simulink model "ES249A_MotAgCorrln"  (R2013b)
settings: Solver=FixedStepDiscrete  SolverMode=SingleTasking  StartTime=0.0  StopTime=1  FixedStep=0.002  RelTol=1e-3
undefined symbols (not defined in the file): FLTINJ_MOTAGCORRLN_MOTAGIDPTSIG, HALFREV_MOTREV_U0P16, MOTAGACORRLNST_CNT_U08, MotAgAMotAgBCorrln, MotAgAMotAgCCorrln, MOTAGBCORRLNST_CNT_U08, MotAgBMotAgCCorrln, MOTAGCCORRLNST_CNT_U08, MOTAGCORRLNERRTHD_MOTREVELEC_U0P16, MOTAGCORRLNNTCFAILSTEP_CNT_U16, MOTAGCORRLNNTCPASSSTEP_CNT_U16, MOTAGMAXSTALLCNTR_CNT_U08, MotAgMeclCorrlnSt, MotAgMeclIdptSig, NtcSts1, sigbuilder_block, SysGlbPrmMotPoleCnt
libraries: simulink x5
(part 4 of 4)

== stateflow chart ES249A_MotAgCorrln/MotAgCorrln/MotAgCorrlnPer1/MotAgA vs MotAgB/SetNtcSts/ISO Fault Debounce Design NOT TO BE IMPLEMENTED IN THIS FDD USED ONLY FOR SIMULATION PURPOSES ==
  note: NTCSTS_PASSD           (0)
      | NTCSTS_FAILD             (1)
      | NTCSTS_PREPASSD   (2)
      | NTCSTS_PREFAILD     (3)
      |
      | SIGQLFR_NORES        (0)
      | SIGQLFR_PASSD         (1)
      | SIGQLFR_FAILD           (2)
  note: Nstep Loop
  note: Pstep Loop
  note: 
  (default) -> (junction 89)
  (junction 89) -> (junction 95) [order 1] : [NtcSts == 3]
  (junction 89) -> (junction 93) [order 2] : [ NtcSts == 2]
  (junction 93) -> (junction 230) [order 2] : {
      | ErrAcc = ErrAcc - DebStep;
      | }
  (junction 95) -> (junction 213) [order 1] : [ErrAcc <=0]
      | {
      | ErrAcc = DebStep;
      | }
  (junction 95) -> (junction 103) [order 2]
  (junction 89) -> (junction 221) [order 3] : [(NtcSts == 0) | ...
      | (NtcSts == 1)]
  (junction 93) -> (junction 123) [order 1] : [(ErrAcc - DebStep) <= -32768]
      | {
      | ErrAcc = -32768;
      | Qualifier = 1;
      | }
  (junction 230) -> (junction 231)
  (junction 213) -> (junction 216)
  (junction 103) -> (junction 216) [order 2] : {
      | ErrAcc = ErrAcc + DebStep;
      | }
  (junction 221) -> (junction 222) [order 2] : [NtcSts == 0]
      | {
      | ErrAcc = -32768;
      | Qualifier=1;
      | }
  (junction 216) -> (junction 214)
  (junction 103) -> (junction 220) [order 1] : [(ErrAcc + DebStep) >=32767]
      | {
      | ErrAcc = 32767;
      | Qualifier =2;
      | }
  (junction 221) -> (junction 212) [order 1] : [NtcSts == 1]
      | {
      | ErrAcc = 32767;
      | Qualifier =2;
      |  }
  (junction 222) -> (junction 225)
  (junction 225) -> (junction 212)
  (junction 212) -> (junction 141)
  (junction 214) -> (junction 220)
  (junction 220) -> (junction 141)
  (junction 123) -> (junction 141)
  (junction 231) -> (junction 123)
  (junction 141) -> (junction 159)
  (junction 159) -> (junction 235) [order 2]
  (junction 235) -> (junction 236)
  (junction 159) -> (junction 234) [order 1] : [SvcClr ==1]
      | {
      | ErrAcc = 0;
      | Qualifier =0;
      | }
  (junction 236) -> (junction 234)
  data: NtcSts input uint8; Qualifier output uint8; DebStep input uint16; ErrAcc output int16; SvcClr input

== matlab function ES249A_MotAgCorrln/MotAgCorrln/MotAgCorrlnPer1/TestOk ==
  data: MotAgAvsMotAgB input boolean; MotAgAOk output boolean; MotAgAvsMotAgC input boolean; MotAgBvsMotAgC input boolean; MotAgBOk output boolean; MotAgCOk output boolean
function [MotAgAOk, MotAgBOk, MotAgCOk] = fcn(MotAgAvsMotAgB, MotAgAvsMotAgC, MotAgBvsMotAgC)

aVarTruthTableCondition_1 = false;
aVarTruthTableCondition_2 = false;
aVarTruthTableCondition_3 = false;


% MotAgAvsMotAgB TestOk

aVarTruthTableCondition_1 = logical(MotAgAvsMotAgB == 1);

% MotAgAvsMotAgC TestOk

aVarTruthTableCondition_2 = logical(MotAgAvsMotAgC == 1);

% MotAgBvsMotAgC TestOk

aVarTruthTableCondition_3 = logical(MotAgBvsMotAgC == 1);

if (aVarTruthTableCondition_1 && aVarTruthTableCondition_2 && aVarTruthTableCondition_3)
    aFcnTruthTableAction_1();
elseif (aVarTruthTableCondition_1 && aVarTruthTableCondition_2 && ~aVarTruthTableCondition_3)
    aFcnTruthTableAction_1();
elseif (aVarTruthTableCondition_1 && ~aVarTruthTableCondition_2 && aVarTruthTableCondition_3)
    aFcnTruthTableAction_1();
elseif (aVarTruthTableCondition_1 && ~aVarTruthTableCondition_2 && ~aVarTruthTableCondition_3)
    aFcnTruthTableAction_2();
elseif (~aVarTruthTableCondition_1 && aVarTruthTableCondition_2 && aVarTruthTableCondition_3)
    aFcnTruthTableAction_1();
elseif (~aVarTruthTableCondition_1 && aVarTruthTableCondition_2 && ~aVarTruthTableCondition_3)
    aFcnTruthTableAction_3();
elseif (~aVarTruthTableCondition_1 && ~aVarTruthTableCondition_2 && aVarTruthTableCondition_3)
    aFcnTruthTableAction_4();
else % Default
    aFcnTruthTableAction_5();
end

function aFcnTruthTableAction_1()

% All good

MotAgAOk = true;
MotAgBOk = true;
MotAgCOk = true;

function aFcnTruthTableAction_2()

% 1 and 2 good

MotAgAOk = true;
MotAgBOk = true;
MotAgCOk = false;

function aFcnTruthTableAction_3()

% 1 and 3 good

MotAgAOk = true;
MotAgBOk = false;
MotAgCOk = true;

function aFcnTruthTableAction_4()

% 2 and 3 good

MotAgAOk = false;
MotAgBOk = true;
MotAgCOk = true;

function aFcnTruthTableAction_5()

% Default (none good)

MotAgAOk = false;
MotAgBOk = false;
MotAgCOk = false;

== stateflow chart ES249A_MotAgCorrln/MotAgCorrln/MotAgCorrlnPer1/MotAgA vs MotAgC/SetNtcSts/ISO Fault Debounce Design NOT TO BE IMPLEMENTED IN THIS FDD USED ONLY FOR SIMULATION PURPOSES ==
  note: NTCSTS_PASSD           (0)
      | NTCSTS_FAILD             (1)
      | NTCSTS_PREPASSD   (2)
      | NTCSTS_PREFAILD     (3)
      |
      | SIGQLFR_NORES        (0)
      | SIGQLFR_PASSD         (1)
      | SIGQLFR_FAILD           (2)
  note: Nstep Loop
  note: Pstep Loop
  note: 
  (default) -> (junction 89)
  (junction 89) -> (junction 95) [order 1] : [NtcSts == 3]
  (junction 89) -> (junction 93) [order 2] : [ NtcSts == 2]
  (junction 93) -> (junction 230) [order 2] : {
      | ErrAcc = ErrAcc - DebStep;
      | }
  (junction 95) -> (junction 213) [order 1] : [ErrAcc <=0]
      | {
      | ErrAcc = DebStep;
      | }
  (junction 95) -> (junction 103) [order 2]
  (junction 89) -> (junction 221) [order 3] : [(NtcSts == 0) | ...
      | (NtcSts == 1)]
  (junction 93) -> (junction 123) [order 1] : [(ErrAcc - DebStep) <= -32768]
      | {
      | ErrAcc = -32768;
      | Qualifier = 1;
      | }
  (junction 230) -> (junction 231)
  (junction 213) -> (junction 216)
  (junction 103) -> (junction 216) [order 2] : {
      | ErrAcc = ErrAcc + DebStep;
      | }
  (junction 221) -> (junction 222) [order 2] : [NtcSts == 0]
      | {
      | ErrAcc = -32768;
      | Qualifier=1;
      | }
  (junction 216) -> (junction 214)
  (junction 103) -> (junction 220) [order 1] : [(ErrAcc+DebStep) >=32767]
      | {
      | ErrAcc = 32767;
      | Qualifier =2;
      | }
  (junction 221) -> (junction 212) [order 1] : [NtcSts == 1]
      | {
      | ErrAcc = 32767;
      | Qualifier =2;
      |  }
  (junction 222) -> (junction 225)
  (junction 225) -> (junction 212)
  (junction 212) -> (junction 141)
  (junction 214) -> (junction 220)
  (junction 220) -> (junction 141)
  (junction 123) -> (junction 141)
  (junction 231) -> (junction 123)
  (junction 141) -> (junction 159)
  (junction 159) -> (junction 235) [order 2]
  (junction 235) -> (junction 236)
  (junction 159) -> (junction 234) [order 1] : [SvcClr ==1]
      | {
      | ErrAcc = 0;
      | Qualifier =0;
      | }
  (junction 236) -> (junction 234)
  data: NtcSts input uint8; Qualifier output uint8; DebStep input uint16; ErrAcc output int16; SvcClr input

== matlab function ES249A_MotAgCorrln/MotAgCorrln/MotAgCorrlnPer1/NotFailed ==
  data: MotAgAvsMotAgB input uint8; MotAgSigAvlA input boolean; MotAgANotFailed output boolean; MotAgAvsMotAgC input uint8; MotAgSigAvlB input boolean; MotAgBvsMotAgC input uint8; MotAgBNotFailed output boolean; MotAgCNotFailed output boolean; MotAgMeclIdptSig output uint8; MotAgSigAvlC input boolean
function [MotAgANotFailed, MotAgBNotFailed, MotAgCNotFailed, MotAgMeclIdptSig] = fcn(MotAgAvsMotAgB, MotAgSigAvlA, MotAgAvsMotAgC, MotAgSigAvlB, MotAgBvsMotAgC, MotAgSigAvlC)

aVarTruthTableCondition_1 = false;
aVarTruthTableCondition_2 = false;
aVarTruthTableCondition_3 = false;


% MotAgAvsMotAgB Not Failed

aVarTruthTableCondition_1 = logical(MotAgAvsMotAgB < 2);

% MotAgAvsMotAgC Not Failed

aVarTruthTableCondition_2 = logical(MotAgAvsMotAgC < 2);

% MotAgBvsMotAgC Not Failed

aVarTruthTableCondition_3 = logical(MotAgBvsMotAgC < 2);

if (aVarTruthTableCondition_1 && aVarTruthTableCondition_2 && aVarTruthTableCondition_3)
    aFcnTruthTableAction_1();
elseif (aVarTruthTableCondition_1 && aVarTruthTableCondition_2 && ~aVarTruthTableCondition_3)
    aFcnTruthTableAction_1();
elseif (aVarTruthTableCondition_1 && ~aVarTruthTableCondition_2 && aVarTruthTableCondition_3)
    aFcnTruthTableAction_1();
elseif (aVarTruthTableCondition_1 && ~aVarTruthTableCondition_2 && ~aVarTruthTableCondition_3)
    aFcnTruthTableAction_2();
elseif (~aVarTruthTableCondition_1 && aVarTruthTableCondition_2 && aVarTruthTableCondition_3)
    aFcnTruthTableAction_1();
elseif (~aVarTruthTableCondition_1 && aVarTruthTableCondition_2 && ~aVarTruthTableCondition_3)
    aFcnTruthTableAction_3();
elseif (~aVarTruthTableCondition_1 && ~aVarTruthTableCondition_2 && aVarTruthTableCondition_3)
    aFcnTruthTableAction_4();
else % Default
    aFcnTruthTableAction_5();
end

function aFcnTruthTableAction_1()

% All good

MotAgANotFailed = true;
MotAgBNotFailed = true;
MotAgCNotFailed = true;
MotAgMeclIdptSig=uint8(MotAgSigAvlA+MotAgSigAvlB+MotAgSigAvlC);

function aFcnTruthTableAction_2()

% 1 and 2 good

MotAgANotFailed = true;
MotAgBNotFailed = true;
MotAgCNotFailed = false;
MotAgMeclIdptSig = uint8(MotAgSigAvlA+MotAgSigAvlB);

function aFcnTruthTableAction_3()

% 1 and 3 good

MotAgANotFailed = true;
MotAgBNotFailed = false;
MotAgCNotFailed = true;
MotAgMeclIdptSig=uint8(MotAgSigAvlA+MotAgSigAvlC);

function aFcnTruthTableAction_4()

% 2 and 3 good

MotAgANotFailed = false;
MotAgBNotFailed = true;
MotAgCNotFailed = true;
MotAgMeclIdptSig=uint8(MotAgSigAvlB+MotAgSigAvlC);

function aFcnTruthTableAction_5()

% Default (none good)

MotAgANotFailed = false;
MotAgBNotFailed = false;
MotAgCNotFailed = false;
MotAgMeclIdptSig = uint8(0);

== stateflow chart ES249A_MotAgCorrln/MotAgCorrln/MotAgCorrlnPer1/MotAgB vs MotAgC/SetNtcSts/ISO Fault Debounce Design NOT TO BE IMPLEMENTED IN THIS FDD USED ONLY FOR SIMULATION PURPOSES ==
  note: NTCSTS_PASSD           (0)
      | NTCSTS_FAILD             (1)
      | NTCSTS_PREPASSD   (2)
      | NTCSTS_PREFAILD     (3)
      |
      | SIGQLFR_NORES        (0)
      | SIGQLFR_PASSD         (1)
      | SIGQLFR_FAILD           (2)
  note: Nstep Loop
  note: Pstep Loop
  note: 
  (default) -> (junction 89)
  (junction 89) -> (junction 95) [order 1] : [NtcSts == 3]
  (junction 89) -> (junction 93) [order 2] : [ NtcSts == 2]
  (junction 93) -> (junction 230) [order 2] : {
      | ErrAcc = ErrAcc - DebStep;
      | }
  (junction 95) -> (junction 213) [order 1] : [ErrAcc <=0]
      | {
      | ErrAcc = DebStep;
      | }
  (junction 95) -> (junction 103) [order 2]
  (junction 89) -> (junction 221) [order 3] : [(NtcSts == 0) | ...
      | (NtcSts == 1)]
  (junction 93) -> (junction 123) [order 1] : [(ErrAcc - DebStep) <= -32768]
      | {
      | ErrAcc = -32768;
      | Qualifier = 1;
      | }
  (junction 230) -> (junction 231)
  (junction 213) -> (junction 216)
  (junction 103) -> (junction 216) [order 2] : {
      | ErrAcc = ErrAcc + DebStep;
      | }
  (junction 221) -> (junction 222) [order 2] : [NtcSts == 0]
      | {
      | ErrAcc = -32768;
      | Qualifier=1;
      | }
  (junction 216) -> (junction 214)
  (junction 103) -> (junction 220) [order 1] : [(ErrAcc + DebStep) >=32767]
      | {
      | ErrAcc = 32767;
      | Qualifier =2;
      | }
  (junction 221) -> (junction 212) [order 1] : [NtcSts == 1]
      | {
      | ErrAcc = 32767;
      | Qualifier =2;
      |  }
  (junction 222) -> (junction 225)
  (junction 225) -> (junction 212)
  (junction 212) -> (junction 141)
  (junction 214) -> (junction 220)
  (junction 220) -> (junction 141)
  (junction 123) -> (junction 141)
  (junction 231) -> (junction 123)
  (junction 141) -> (junction 159)
  (junction 159) -> (junction 235) [order 2]
  (junction 235) -> (junction 236)
  (junction 159) -> (junction 234) [order 1] : [SvcClr ==1]
      | {
      | ErrAcc = 0;
      | Qualifier =0;
      | }
  (junction 236) -> (junction 234)
  data: NtcSts input uint8; Qualifier output uint8; DebStep input uint16; ErrAcc output int16; SvcClr input

== stateflow chart ES249A_MotAgCorrln/MotAgCorrln/MotAgCorrlnPer1/MtrAgC SigAvlCheck/CorrSigAvlChkRev1 ==
  note: SigAvl
      | False = 0
      | Pass = 1
  note: SigQlfr
      | 0 = No Result
      | 1 = Pass
      | 2 = Fail
  (default) -> (junction 2)
  (junction 2) -> (junction 4) [order 1] : [SigRollgCnt ==LstRollgCnt]
  (junction 4) -> (junction 7) [order 2] : {
      | StallCntOutp = LstStallCnt +1;
      | }
  (junction 2) -> (junction 3) [order 2]
  (junction 4) -> (junction 7) [order 1] : [LstStallCnt == 255]
      | {
      | StallCntOutp = 255;
      | }
  (junction 3) -> (junction 7) : {
      | StallCntOutp = 0;
      | }
  (junction 7) -> (junction 10)
  (junction 10) -> (junction 12) [order 1] : [StallCntOutp >=kMaxStallCnt]
  (junction 10) -> (junction 14) [order 2]
  (junction 12) -> (junction 17)
  (junction 14) -> (junction 17) [order 2]
  (junction 14) -> (junction 16) [order 1] : [SigQlfr<2]
  (junction 17) -> (junction 29) : {
      | SigAvl =0;
      | }
  (junction 16) -> (junction 29) : {
      | SigAvl = 1;
      | }
  data: SigRollgCnt input; SigQlfr input; kMaxStallCnt input; SigAvl output boolean; LstRollgCnt input uint8; LstStallCnt input uint8; StallCntOutp output uint8

== stateflow chart ES249A_MotAgCorrln/MotAgCorrln/MotAgCorrlnPer1/MtrAgB SigAvlCheck/CorrSigAvlChkRev1 ==
  note: SigAvl
      | False = 0
      | Pass = 1
  note: SigQlfr
      | 0 = No Result
      | 1 = Pass
      | 2 = Fail
  (default) -> (junction 2)
  (junction 2) -> (junction 4) [order 1] : [SigRollgCnt ==LstRollgCnt]
  (junction 4) -> (junction 7) [order 2] : {
      | StallCntOutp = LstStallCnt +1;
      | }
  (junction 2) -> (junction 3) [order 2]
  (junction 4) -> (junction 7) [order 1] : [LstStallCnt == 255]
      | {
      | StallCntOutp = 255;
      | }
  (junction 3) -> (junction 7) : {
      | StallCntOutp = 0;
      | }
  (junction 7) -> (junction 10)
  (junction 10) -> (junction 12) [order 1] : [StallCntOutp >=kMaxStallCnt]
  (junction 10) -> (junction 14) [order 2]
  (junction 12) -> (junction 17)
  (junction 14) -> (junction 17) [order 2]
  (junction 14) -> (junction 16) [order 1] : [SigQlfr<2]
  (junction 17) -> (junction 29) : {
      | SigAvl =0;
      | }
  (junction 16) -> (junction 29) : {
      | SigAvl = 1;
      | }
  data: SigRollgCnt input; SigQlfr input; kMaxStallCnt input; SigAvl output boolean; LstRollgCnt input uint8; LstStallCnt input uint8; StallCntOutp output uint8

== stateflow chart ES249A_MotAgCorrln/MotAgCorrln/MotAgCorrlnPer1/MtrAgA SigAvlCheck/CorrSigAvlChkRev1 ==
  note: SigAvl
      | False = 0
      | Pass = 1
  note: SigQlfr
      | 0 = No Result
      | 1 = Pass
      | 2 = Fail
  (default) -> (junction 2)
  (junction 2) -> (junction 4) [order 1] : [SigRollgCnt ==LstRollgCnt]
  (junction 4) -> (junction 7) [order 2] : {
      | StallCntOutp = LstStallCnt +1;
      | }
  (junction 2) -> (junction 3) [order 2]
  (junction 4) -> (junction 7) [order 1] : [LstStallCnt == 255]
      | {
      | StallCntOutp = 255;
      | }
  (junction 3) -> (junction 7) : {
      | StallCntOutp = 0;
      | }
  (junction 7) -> (junction 10)
  (junction 10) -> (junction 12) [order 1] : [StallCntOutp >=kMaxStallCnt]
  (junction 10) -> (junction 14) [order 2]
  (junction 12) -> (junction 17)
  (junction 14) -> (junction 17) [order 2]
  (junction 14) -> (junction 16) [order 1] : [SigQlfr<2]
  (junction 17) -> (junction 29) : {
      | SigAvl =0;
      | }
  (junction 16) -> (junction 29) : {
      | SigAvl = 1;
      | }
  data: SigRollgCnt input; SigQlfr input; kMaxStallCnt input; SigAvl output boolean; LstRollgCnt input uint8; LstStallCnt input uint8; StallCntOutp output uint8
